simulink model "tp4ejercicio10b"  (R2021a)
settings: Solver=VariableStepAuto  StartTime=0.0  StopTime=10.0  RelTol=1e-3
undefined symbols (not defined in the file or in its folder): gray, Rec, SDTV
libraries: visionconversions x2, visionsources x1
settings Model: Creator=ZeK005  LastModifiedBy=ZeK005

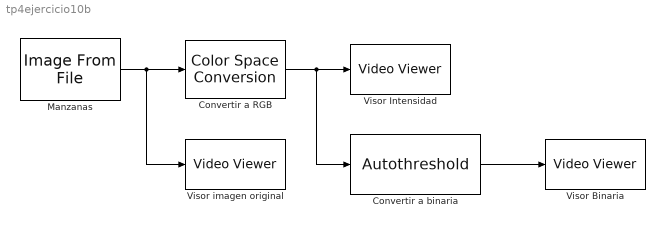
== system tp4ejercicio10b ==
  Convertir a RGB : visionconversions/Color Space  Conversion  conversion=Obsolete  conversionActive=R'G'B' to intensity  wp_str=D65  rec=Rec. 601 (SDTV)  sys=1125/60/2:1  imagePorts=One multidimensional signal
  Convertir a binaria : visionconversions/Autothreshold  operator=>  threshOut=off  effMetricOut=off  userDefinedRange=off  umin=0  umax=255  outOfRngOpt=Ignore  scaleThreshold=off  scaleFactor=1  roundingMode=Floor  overflowMode=off  P1Mode=Specify word length  P1WordLength=32  P1FracLength=30  P2Mode=Specify word length  P2WordLength=32  P2FracLength=22  P3Mode=Specify word length  P3WordLength=32  P3FracLength=14  P4Mode=Binary point scaling  P4WordLength=32  P4FracLength=15  Q1Mode=Specify word length  Q1WordLength=32  Q1FracLength=16  EMMode=Specify word length  EMWordLength=16  EMFracLength=14
      settings: SourceProductBaseCode=VP
  Manzanas : visionsources/Image From File  Tag=vipblks_nd  FileName=C:\Users\ZeK005\Desktop\FRT UTN\Proyectos\Matlab\2024\PDI\manzanas.jpg  Ts=inf  imagePorts=One multidimensional signal  OutPortLabels=R|G|B  ImageDataType=Inherit from input image  sdImageDataType=uint(8)  Signed=on  WordLength=16  FractionLengthMode=User-defined  FractionLength=15
  Visor Binaria : VideoViewer  colormapValue=gray(256)  FigPos=[638 872 666 405]
  Visor Intensidad : VideoViewer  colormapValue=gray(256)  FigPos=[73 853 666 405]
  Visor imagen original : VideoViewer  colormapValue=gray(256)  FigPos=[967 883 666 405]
  wires:
  Manzanas/1 -> Visor imagen original/1, Convertir a RGB/1
  Convertir a RGB/1 -> Convertir a binaria/1, Visor Intensidad/1
  Convertir a binaria/1 -> Visor Binaria/1
